simulink model "SAS_Flaperon_F35_FullModel_v1"  (R2025b)
settings: Solver=ode15s  StartTime=0.0  StopTime=10.0  RelTol=1e-3
settings Model: Creator=ikita  LastModifiedBy=mikol

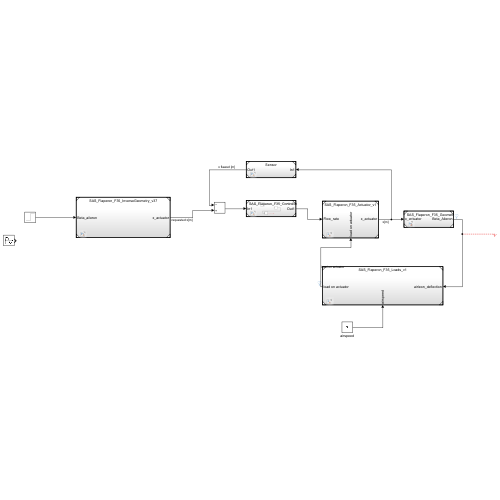
[thumbnail: Simulink's stored preview of the top-level diagram]
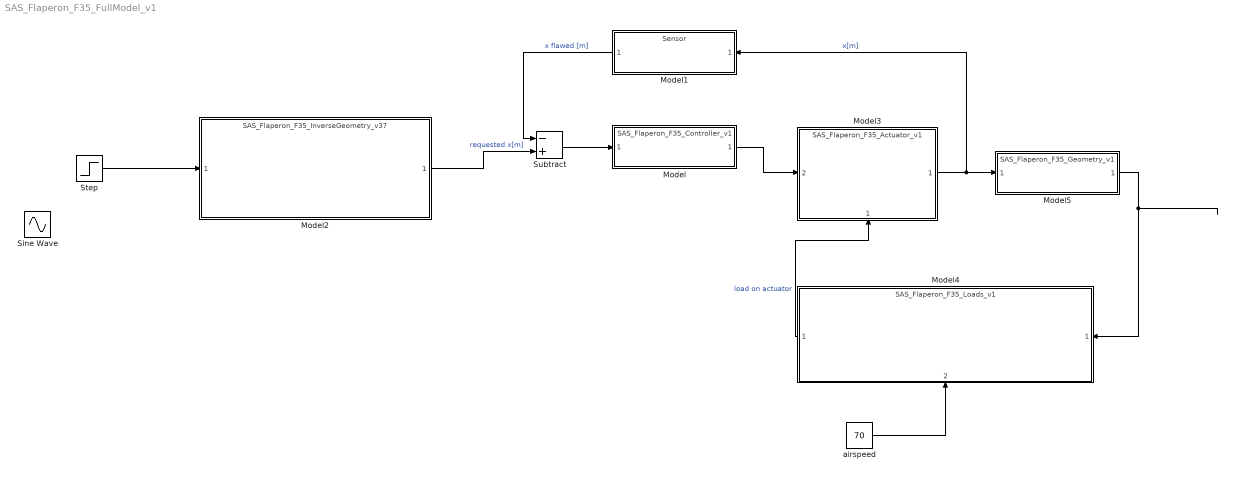
== system SAS_Flaperon_F35_FullModel_v1 ==
  Model : ModelReference  ModelNameDialog=SAS_Flaperon_F35_Controller_v1.slx  SimulationMode=Normal  ModelReferenceVersion=1.19
  Model1 : ModelReference  ModelNameDialog=Sensor.slx  SimulationMode=Normal  ModelReferenceVersion=1.3
  Model2 : ModelReference  ModelNameDialog=SAS_Flaperon_F35_InverseGeometry_v37  SimulationMode=Normal  ModelReferenceVersion=1.7
  Model3 : ModelReference  ModelNameDialog=SAS_Flaperon_F35_Actuator_v1  SimulationMode=Normal  ModelReferenceVersion=1.11
      settings: PortSchema="{\"entries\":[{\"content\":{\"sides\":[{\"content\":{\"connectorIds\":[\"In2\"]},\"type\":\"ConnectorPlacement.EquallySpacedRectSide\",\"uuid\":\"b3fa62ef-1018-4006-82f9-e4f5866ce4fe\"},{\"content\":{\"connectorIds\":[\"Out1\"],\"side\":\"RIGHT\"},\"type\":\"ConnectorPlacement.EquallySpacedRectSide\",\"uuid\":\"ffe0a412-f91f-42cd-838e-8f28da290aba\"},{\"content\":{\"side\":\"TOP\"},\"type\":\"ConnectorPlacement.EquallySpacedRectSide\",\"uuid\":\"6e6c5404-7aaa-4007-9cca-ac77abd891dd\"},{\"content\":{\"connectorIds\":[\"In1\"],\"side\":\"BOTTOM\"},\"type\":\"ConnectorPlacement.EquallySpacedRectSide\",\"uuid\":\"7ed0818f-e9ce-427c-b423-a2a3263b756f\"}]},\"type\":\"ConnectorPlacement.EquallySpacedConnector\",\"uuid\":\"e9fd68ea-2f1d-4e03-98ba-4a3a3c65fe2d\"}],\"packageUris\":[\"http://schema.mathworks.com/mf0/Connector/R2020b\"],\"version\":\"1.0\"}"
  Model4 : ModelReference  ModelNameDialog=SAS_Flaperon_F35_Loads_v1  SimulationMode=Normal  ModelReferenceVersion=1.8
      settings: PortSchema="{\"entries\":[{\"content\":{\"sides\":[{\"content\":{\"connectorIds\":[\"In1\"]},\"type\":\"ConnectorPlacement.EquallySpacedRectSide\",\"uuid\":\"1e434847-8d43-4bcd-b697-9d66e26c93f9\"},{\"content\":{\"connectorIds\":[\"Out1\"],\"side\":\"RIGHT\"},\"type\":\"ConnectorPlacement.EquallySpacedRectSide\",\"uuid\":\"60552336-a692-4697-8576-8ac7d0ff8a44\"},{\"content\":{\"side\":\"TOP\"},\"type\":\"ConnectorPlacement.EquallySpacedRectSide\",\"uuid\":\"31f5c284-40ed-40a6-9600-b515867fc2ae\"},{\"content\":{\"connectorIds\":[\"In2\"],\"side\":\"BOTTOM\"},\"type\":\"ConnectorPlacement.EquallySpacedRectSide\",\"uuid\":\"5ff11c7b-acb7-4f0e-b186-e6c027e78aca\"}]},\"type\":\"ConnectorPlacement.EquallySpacedConnector\",\"uuid\":\"9cd4bfca-3652-473e-9b0a-d6647edae380\"}],\"packageUris\":[\"http://schema.mathworks.com/mf0/Connector/R2020b\"],\"version\":\"1.0\"}"
  Model5 : ModelReference  ModelNameDialog=SAS_Flaperon_F35_Geometry_v1  SimulationMode=Normal  ModelReferenceVersion=1.7
  Sine Wave : Sin  Amplitude=25  Frequency=0.5  SampleTime=0
  Step : Step  After=30  SampleTime=0
  Subtract : Sum  Inputs=-+
  airspeed : Constant  Value=70
  wires:
  Subtract/1 -> Model/1
  Model1/1 -> Subtract/1  "x flawed [m]"
  Model3/1 -> Model1/1, Model5/1  "x[m]"
  Model5/1 -> Model4/1
  airspeed/1 -> Model4/2
  Model4/1 -> Model3/1  "load on actuator"
  Model2/1 -> Subtract/2  "requested x[m]"
  Model/1 -> Model3/2
  Step/1 -> Model2/1
